simulink model "momentumBasedFlightSim"  (R2022a)
settings: Solver=FixedStepDiscrete  StartTime=0.0  StopTime=Config.simulationTime  FixedStep=Config.tStep  RelTol=1e-3
InitFcn:
  | cd(fileparts(which(bdroot)));
  | initMomentumBasedFlight;
StopFcn:
  | cd(fileparts(which(bdroot)));
  | stopMomentumBasedFlight;
undefined symbols (not defined in the file or in its folder): Config, DiscIntNeverNeededParam
libraries: WBToolboxLibrary x31, cstblocks x3, momentum_flight_control_sublib x2, thrust_estimation_sublib x1, jets_control x1
(part 2 of 2)

== system momentumBasedFlightSim/FLIGHT CONTROLLER (CORE) V6.0/FLIGHT CONTROL/Momentum-based Flight Control QP/Filtering and Saturations/Filters on jointVel ==
  jointVel_star_QP : Inport
  Compare_filtered_jointVel : Scope  NumInputPorts=2
  Constant : Constant  Value=ones(4,1)*11
  Constant1 : Constant  Value=Config.BALANCING_NO_JETS
  Constant2 : Constant  Value=Config.filter.cutOffFrequency
  Constant3 : Constant  Value=Config.FILTER_SDOT_AFTER_QP
  Dead Zone1 : DeadZone  LowerValue=-Config.deadzone.jointVel_deadzone  UpperValue=Config.deadzone.jointVel_deadzone
  Discrete Varying Lowpass1 : cstblocks/Linear Parameter Varying/Discrete Varying Lowpass  N=2  w0=0  Ts=Config.tStep
      settings: SourceProductBaseCode=CT
  Saturation1 : Saturate  UpperLimit=Config.saturation.maxJointVelDes  LowerLimit=-Config.saturation.maxJointVelDes
  Switch : Switch  Criteria=u2 > Threshold  SaturateOnIntegerOverflow=off  InputSameDT=off
  Switch1 : Switch  Criteria=u2 > Threshold  SaturateOnIntegerOverflow=off  InputSameDT=off
  joint_vel_saturation : MATLAB Function  TreatAsAtomicUnit=on
  jointVel_star_filt : Outport  VectorParamsAs1DForOutWhenUnconnected=off
  tag scope: JointVelocityDesired=global
  wires:
  Constant3/1 -> Switch1/2
  Switch1/1 -> jointVel_star_filt/1
  joint_vel_saturation/1(jointVel) -> Switch1/1, Compare_filtered_jointVel/1
  Constant2/1 -> Discrete Varying Lowpass1/2
  Saturation1/1 -> joint_vel_saturation/2(jointVel_des)
  Discrete Varying Lowpass1/1 -> Dead Zone1/1
  Dead Zone1/1 -> Saturation1/1
  jointVel_star_QP/1 -> Discrete Varying Lowpass1/1, Switch1/3, Compare_filtered_jointVel/2, [JointVelocityDesired]
  Switch/1 -> joint_vel_saturation/3(JetState)
  Constant1/1 -> Switch/2
  [JetLog] -> Switch/3
  Constant/1 -> Switch/1
  [jointPos_meas] -> joint_vel_saturation/1(jointPos)

== system momentumBasedFlightSim/FLIGHT CONTROLLER (CORE) V6.0/FLIGHT CONTROL/Flight 0 Reference Generator/Compute Gains And References/Online Planner/Smooth CoM References ==
  posCoM_des : Inport
  accCoM_gravity_ref : Inport  Port=2
  Combine CoM References : MATLAB Function  TreatAsAtomicUnit=on
  MatchSignalSizes{,1..3} (4 alike) : WBToolboxLibrary/Utilities/MatchSignalSizes
      settings: SourceProductName=WholeBodyToolbox
  MinimumJerkTrajectoryGenerator : WBToolboxLibrary/Utilities/MinimumJerkTrajectoryGenerator  externalSettlingTime=off  settlingTime=Config.planner.timeToReachHovering  sampleTime=Config.tStep  resetOnSettlingTime=off  firstDerivatives=off  secondDerivatives=off  explicitInitialValue=off
      settings: SourceProductName=WholeBodyToolbox
  MinimumJerkTrajectoryGenerator1 : WBToolboxLibrary/Utilities/MinimumJerkTrajectoryGenerator  externalSettlingTime=off  settlingTime=Config.planner.smoothingTimeCoMRef  sampleTime=Config.tStep  resetOnSettlingTime=off  firstDerivatives=on  secondDerivatives=on  explicitInitialValue=off
      settings: SourceProductName=WholeBodyToolbox
  pos_vel_acc_jerk_CoM_des : Outport  VectorParamsAs1DForOutWhenUnconnected=off
  wires:
  MinimumJerkTrajectoryGenerator/1 -> MatchSignalSizes3/2
  MinimumJerkTrajectoryGenerator1/3 -> MatchSignalSizes2/2
  MinimumJerkTrajectoryGenerator1/2 -> MatchSignalSizes1/2
  posCoM_des/1 -> MinimumJerkTrajectoryGenerator1/1, MatchSignalSizes1/1, MatchSignalSizes2/1, MatchSignalSizes3/1, MatchSignalSizes/1
  MatchSignalSizes1/1 -> Combine CoM References/2(CoM_vel)
  MatchSignalSizes2/1 -> Combine CoM References/3(CoM_acc)
  MatchSignalSizes3/1 -> Combine CoM References/4(CoM_acc_gravity)
  MatchSignalSizes/1 -> Combine CoM References/1(CoM_pos)
  MinimumJerkTrajectoryGenerator1/1 -> MatchSignalSizes/2
  accCoM_gravity_ref/1 -> MinimumJerkTrajectoryGenerator/1
  Combine CoM References/1(pos_vel_acc_jerk_CoM_des) -> pos_vel_acc_jerk_CoM_des/1

== system momentumBasedFlightSim/FLIGHT CONTROLLER (CORE) V6.0/FLIGHT CONTROL/Momentum-based Flight Control QP/Compute QP Quantities/Integrate CoM Velocity/Get CoM Position Error from Integral ==
  kinematics : Inport
  systemState : Inport  Port=2
  gainsAndReferences : Inport  Port=3
  Bus Selector : BusSelector  OutputSignals=stateVel
  Bus Selector1 : BusSelector  OutputSignals=pos_vel_acc_jerk_CoM_des
  Bus Selector2 : BusSelector  OutputSignals=J_CoM
  Constant : Constant  Value=zeros(3,1)
  Dead Zone : DeadZone  LowerValue=-Config.deadzone.velCoM_deadzone  UpperValue=Config.deadzone.velCoM_deadzone
  Integrate velCoM_error : DiscreteIntegrator  InitialConditionSource=external  SampleTime=Config.tStep  ICPrevOutput=DiscIntNeverNeededParam  ICPrevScaledInput=DiscIntNeverNeededParam
  MatrixMultiply : Product  Multiplication=Matrix(*)
  Selector1 : Selector  NumberOfDimensions=2  InputPortWidth=3  IndexOptions=Index vector (dialog),Index vector (dialog)  Indices=[1 2 3],2  OutputSizes=1,1
  Sum1 : Sum  Inputs=|+-
  posCoM_error_fromIntegral : Outport
  wires:
  Bus Selector2/1 -> MatrixMultiply/1  "<J_CoM>"
  Selector1/1 -> Sum1/2  "velCoM_des"
  MatrixMultiply/1 -> Sum1/1  "velCoM"
  Integrate velCoM_error/1 -> posCoM_error_fromIntegral/1
  Bus Selector1/1 -> Selector1/1  "<pos_vel_acc_jerk_CoM_des>"
  gainsAndReferences/1 -> Bus Selector1/1
  systemState/1 -> Bus Selector/1
  Sum1/1 -> Dead Zone/1
  kinematics/1 -> Bus Selector2/1
  Bus Selector/1 -> MatrixMultiply/2  "<stateVel>"
  Constant/1 -> Integrate velCoM_error/2
  Dead Zone/1 -> Integrate velCoM_error/1

== system momentumBasedFlightSim/FLIGHT CONTROLLER (CORE) V6.0/FLIGHT CONTROL/Momentum-based Flight Control QP/Compute QP Quantities/Integrate CoM Velocity/Get CoM Position Error from Integral but Only in Hovering ==
  feetContactIsActive : Inport
  kinematics : Inport  Port=2
  systemState : Inport  Port=3
  gainsAndReferences : Inport  Port=4
  Bus Selector : BusSelector  OutputSignals=stateVel
  Bus Selector1 : BusSelector  OutputSignals=pos_vel_acc_jerk_CoM_des
  Bus Selector2 : BusSelector  OutputSignals=posCoM,J_CoM
  Dead Zone : DeadZone  LowerValue=-Config.deadzone.velCoM_deadzone  UpperValue=Config.deadzone.velCoM_deadzone
  Get CoM initial condition : MATLAB Function  TreatAsAtomicUnit=on
  Integrate velCoM_error : DiscreteIntegrator  ExternalReset=either  InitialConditionSource=external  SampleTime=Config.tStep  ICPrevOutput=DiscIntNeverNeededParam  ICPrevScaledInput=DiscIntNeverNeededParam
  MatrixMultiply : Product  Multiplication=Matrix(*)
  Selector1 : Selector  NumberOfDimensions=2  InputPortWidth=3  IndexOptions=Index vector (dialog),Index vector (dialog)  Indices=[1 2 3],2  OutputSizes=1,1
  Selector2 : Selector  NumberOfDimensions=2  InputPortWidth=3  IndexOptions=Index vector (dialog),Index vector (dialog)  Indices=[1 2 3],1  OutputSizes=1,1
  Sum1 : Sum  Inputs=|+-
  Sum2 : Sum  Inputs=|+-
  Switch : Switch  Criteria=u2 > Threshold  SaturateOnIntegerOverflow=off  InputSameDT=off
  posCoM_error_fromInt_HoveringOnly : Outport
  wires:
  Get CoM initial condition/1(error_posCoM_0) -> Integrate velCoM_error/3
  Bus Selector2/2 -> MatrixMultiply/1  "<J_CoM>"
  Selector1/1 -> Sum1/2  "velCoM_des"
  MatrixMultiply/1 -> Sum1/1  "velCoM"
  Bus Selector1/1 -> Selector2/1, Selector1/1  "<pos_vel_acc_jerk_CoM_des>"
  gainsAndReferences/1 -> Bus Selector1/1
  systemState/1 -> Bus Selector/1
  Sum1/1 -> Dead Zone/1
  kinematics/1 -> Bus Selector2/1
  Bus Selector/1 -> MatrixMultiply/2  "<stateVel>"
  Sum2/1 -> Get CoM initial condition/2(error_posCoM), Switch/1
  Switch/1 -> posCoM_error_fromInt_HoveringOnly/1
  Bus Selector2/1 -> Sum2/1  "<posCoM>"
  Selector2/1 -> Sum2/2  "posCoM_des"
  Integrate velCoM_error/1 -> Switch/3
  feetContactIsActive/1 -> Switch/2, Integrate velCoM_error/2, Get CoM initial condition/1(feetContactIsActive)
  Dead Zone/1 -> Integrate velCoM_error/1

== system momentumBasedFlightSim/FLIGHT CONTROLLER (CORE) V6.0/FLIGHT CONTROL/Momentum-based Flight Control QP/Compute QP Quantities/Integrate CoM Velocity/Get CoM Position Error from Kinematics ==
  kinematics : Inport
  gainsAndReferences : Inport  Port=2
  Bus Selector1 : BusSelector  OutputSignals=pos_vel_acc_jerk_CoM_des
  Bus Selector2 : BusSelector  OutputSignals=posCoM
  Selector1 : Selector  NumberOfDimensions=2  InputPortWidth=3  IndexOptions=Index vector (dialog),Index vector (dialog)  Indices=[1 2 3],1  OutputSizes=1,1
  Sum1 : Sum  Inputs=|+-
  posCoM_error_fromKinematics : Outport
  wires:
  Bus Selector2/1 -> Sum1/1  "<posCoM>"
  Selector1/1 -> Sum1/2  "posCoM_des"
  Sum1/1 -> posCoM_error_fromKinematics/1
  Bus Selector1/1 -> Selector1/1  "<pos_vel_acc_jerk_CoM_des>"
  gainsAndReferences/1 -> Bus Selector1/1
  kinematics/1 -> Bus Selector2/1

== system momentumBasedFlightSim/FLIGHT CONTROLLER (CORE) V6.0/FLIGHT CONTROL/Momentum-based Flight Control QP/Compute QP Quantities/Integrate CoM Velocity/Select CoM Pos Error ==
  feetContactIsActive : Inport
  posCoM_error_fromInt_HoveringOnly : Inport  Port=2
  posCoM_error_fromIntegral : Inport  Port=3
  posCoM_error_fromKinematics : Inport  Port=4
  CoM Pos Errors : Scope  NumInputPorts=4
  Select CoM Pos Error : MATLAB Function  TreatAsAtomicUnit=on
  posCoM_error : Outport
  wires:
  posCoM_error_fromKinematics/1 -> CoM Pos Errors/3, Select CoM Pos Error/3(posCoM_error_fromKinematics)  "posCoM_error_fromKinematics"
  posCoM_error_fromIntegral/1 -> Select CoM Pos Error/2(posCoM_error_fromIntegral), CoM Pos Errors/2  "posCoM_error_fromIntegral"
  posCoM_error_fromInt_HoveringOnly/1 -> CoM Pos Errors/1, Select CoM Pos Error/1(posCoM_error_fromInt_HoveringOnly)  "posCoM_error_fromInt_HoveringOnly"
  Select CoM Pos Error/1(posCoM_error) -> posCoM_error/1
  feetContactIsActive/1 -> CoM Pos Errors/4  "robotIsBalancing"

== system momentumBasedFlightSim/FLIGHT CONTROLLER (CORE) V6.0/FLIGHT CONTROL/Momentum-based Flight Control QP/Compute QP Quantities/Visualize QP Quantities/Cost Function ==
  uStar : Inport
  Hessian : Inport  Port=2
  gradient : Inport  Port=3
  costVectorQP : Inport  Port=4
  Add1 : Sum
  Demux : Demux  Outputs=8
  Full Cost Check : Scope
  Gain : Gain  Gain=0.5
  Matrix Multiply : Product  Multiplication=Matrix(*)
  Matrix Multiply1 : Product  Multiplication=Matrix(*)
  Matrix Multiply2 : Product  Multiplication=Matrix(*)
  Transpose : Math  Operator=transpose
  costs in QP function : Scope  NumInputPorts=8
  wires:
  Demux/1 -> costs in QP function/1  "linMom_xy"
  Gain/1 -> Add1/2  "(uT * H * u) / 2"
  Add1/1 -> Full Cost Check/1  "(uT * H * u)/2 + uT * g"
  gradient/1 -> Matrix Multiply2/2
  Matrix Multiply2/1 -> Add1/1  "uT * g"
  Matrix Multiply1/1 -> Gain/1
  Matrix Multiply/1 -> Matrix Multiply1/1
  Hessian/1 -> Matrix Multiply/2
  Transpose/1 -> Matrix Multiply/1, Matrix Multiply2/1
  uStar/1 -> Transpose/1, Matrix Multiply1/2
  Demux/7 -> costs in QP function/7  "TDotPost"
  Demux/6 -> costs in QP function/6  "legsPost"
  Demux/5 -> costs in QP function/5  "armsPost"
  Demux/2 -> costs in QP function/2  "linMom_z"
  Demux/8 -> costs in QP function/8  "symmTDot"
  Demux/3 -> costs in QP function/3  "angMom"
  Demux/4 -> costs in QP function/4  "torsoPost"
  costVectorQP/1 -> Demux/1

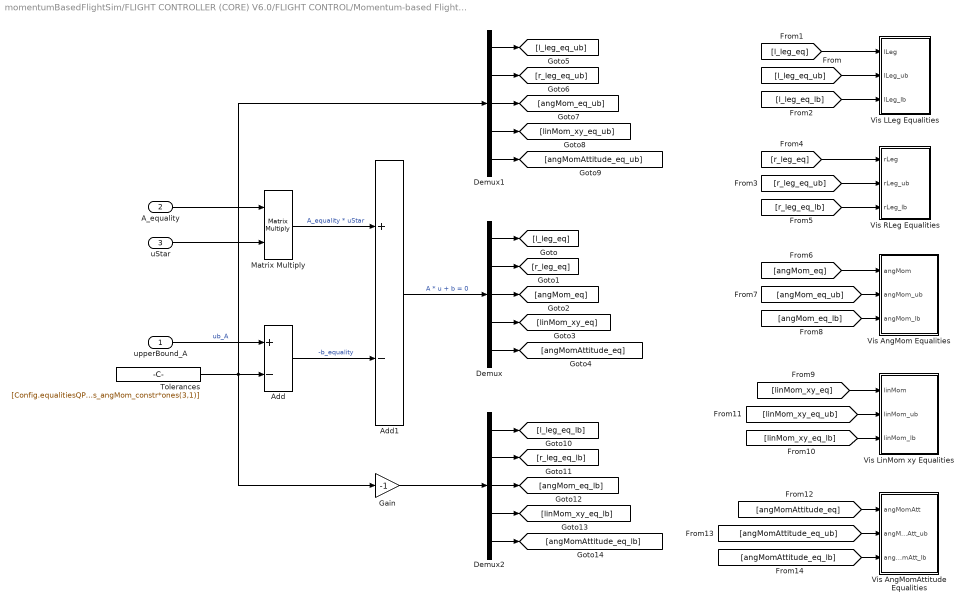
== system momentumBasedFlightSim/FLIGHT CONTROLLER (CORE) V6.0/FLIGHT CONTROL/Momentum-based Flight Control QP/Compute QP Quantities/Visualize QP Quantities/Equality Constraints ==
  upperBound_A : Inport
  A_equality : Inport  Port=2
  uStar : Inport  Port=3
  Add : Sum  Inputs=+-
  Add1 : Sum  Inputs=+-
  Demux : Demux  Outputs=[Config.N_LEGS/2; Config.N_LEGS/2; 3; 2; 3]
  Demux1 : Demux  Outputs=[Config.N_LEGS/2; Config.N_LEGS/2; 3; 2; 3]
  Demux2 : Demux  Outputs=[Config.N_LEGS/2; Config.N_LEGS/2; 3; 2; 3]
  Gain : Gain  Gain=-1
  Matrix Multiply : Product  Multiplication=Matrix(*)
  Tolerances : Constant  Value=[Config.equalitiesQP.eps_legs*ones(Config.N_LEGS,1); Config.equalitiesQP.eps_angMom*ones(3,1); Config.equalitiesQP.eps_linMom_xy*ones(2,1); Config.equalitiesQP.eps_angMom_constr*ones(3,1)]
  Vis AngMom Equalities : Subsystem
  Vis AngMomAttitude Equalities : Subsystem
  Vis LLeg Equalities : Subsystem
  Vis LinMom xy Equalities : Subsystem
  Vis RLeg Equalities : Subsystem
  wires:
  [angMomAttitude_eq_lb] -> Vis AngMomAttitude Equalities/3(angMomAtt_lb)
  [angMomAttitude_eq_ub] -> Vis AngMomAttitude Equalities/2(angMomAtt_ub)
  [angMomAttitude_eq] -> Vis AngMomAttitude Equalities/1(angMomAtt)
  [linMom_xy_eq] -> Vis LinMom xy Equalities/1(linMom)
  [linMom_xy_eq_ub] -> Vis LinMom xy Equalities/2(linMom_ub)
  [linMom_xy_eq_lb] -> Vis LinMom xy Equalities/3(linMom_lb)
  [angMom_eq_lb] -> Vis AngMom Equalities/3(angMom_lb)
  [angMom_eq_ub] -> Vis AngMom Equalities/2(angMom_ub)
  [angMom_eq] -> Vis AngMom Equalities/1(angMom)
  [r_leg_eq_lb] -> Vis RLeg Equalities/3(rLeg_lb)
  [r_leg_eq] -> Vis RLeg Equalities/1(rLeg)
  [r_leg_eq_ub] -> Vis RLeg Equalities/2(rLeg_ub)
  [l_leg_eq_lb] -> Vis LLeg Equalities/3(lLeg_lb)
  [l_leg_eq_ub] -> Vis LLeg Equalities/2(lLeg_ub)
  [l_leg_eq] -> Vis LLeg Equalities/1(lLeg)
  Demux2/1 -> [l_leg_eq_lb]
  Demux2/2 -> [r_leg_eq_lb]
  Demux2/5 -> [angMomAttitude_eq_lb]
  Demux2/4 -> [linMom_xy_eq_lb]
  Demux2/3 -> [angMom_eq_lb]
  Demux1/4 -> [linMom_xy_eq_ub]
  Demux1/2 -> [r_leg_eq_ub]
  Demux1/1 -> [l_leg_eq_ub]
  Demux1/3 -> [angMom_eq_ub]
  Demux1/5 -> [angMomAttitude_eq_ub]
  Demux/5 -> [angMomAttitude_eq]
  Demux/4 -> [linMom_xy_eq]
  Demux/3 -> [angMom_eq]
  Demux/2 -> [r_leg_eq]
  Demux/1 -> [l_leg_eq]
  Tolerances/1 -> Demux1/1, Gain/1, Add/2
  Add1/1 -> Demux/1  "A * u + b = 0"
  Matrix Multiply/1 -> Add1/1  "A_equality * uStar"
  uStar/1 -> Matrix Multiply/2
  A_equality/1 -> Matrix Multiply/1
  Add/1 -> Add1/2  "-b_equality"
  upperBound_A/1 -> Add/1  "ub_A"
  Gain/1 -> Demux2/1

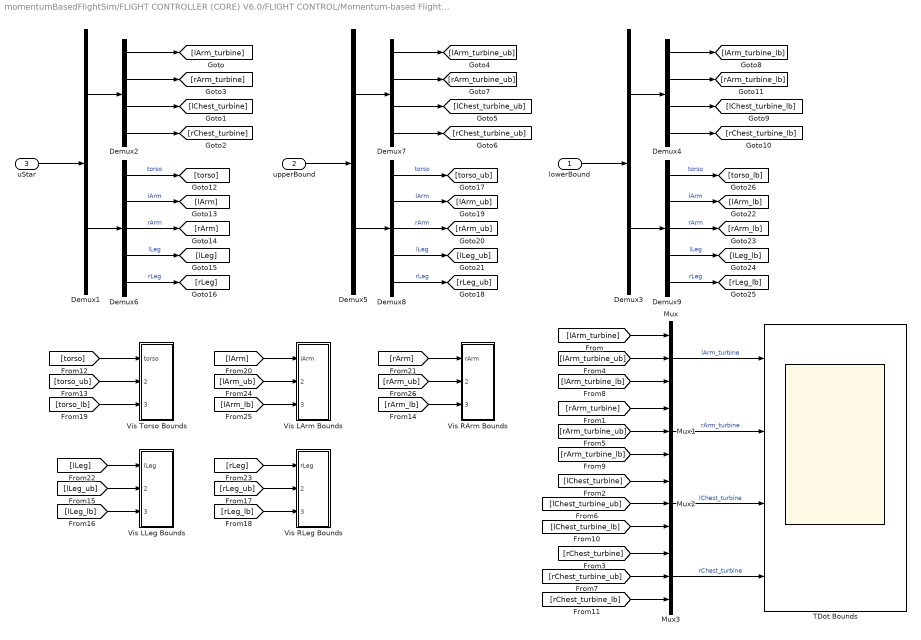
== system momentumBasedFlightSim/FLIGHT CONTROLLER (CORE) V6.0/FLIGHT CONTROL/Momentum-based Flight Control QP/Compute QP Quantities/Visualize QP Quantities/Input Boundaries ==
  lowerBound : Inport
  upperBound : Inport  Port=2
  uStar : Inport  Port=3
  Demux1 : Demux  Outputs=[Config.N_JETS; Config.N_DOF]
  Demux2 : Demux  Outputs=Config.N_JETS
  Demux3 : Demux  Outputs=[Config.N_JETS; Config.N_DOF]
  Demux4 : Demux  Outputs=Config.N_JETS
  Demux5 : Demux  Outputs=[Config.N_JETS; Config.N_DOF]
  Demux6 : Demux  Outputs=Config.numOfJointsForEachControlboard
  Demux7 : Demux  Outputs=Config.N_JETS
  Demux8 : Demux  Outputs=Config.numOfJointsForEachControlboard
  Demux9 : Demux  Outputs=Config.numOfJointsForEachControlboard
  Mux{,1..3} (4 alike) : Mux  Inputs=3
  TDot Bounds : Scope  NumInputPorts=4
  Vis LArm Bounds : Subsystem
  Vis LLeg Bounds : Subsystem
  Vis RArm Bounds : Subsystem
  Vis RLeg Bounds : Subsystem
  Vis Torso Bounds : Subsystem
  wires:
  Mux3/1 -> TDot Bounds/4  "rChest_turbine"
  Mux2/1 -> TDot Bounds/3  "lChest_turbine"
  Mux1/1 -> TDot Bounds/2  "rArm_turbine"
  Mux/1 -> TDot Bounds/1  "lArm_turbine"
  [torso_lb] -> Vis Torso Bounds/3(torso_lb)
  [torso_ub] -> Vis Torso Bounds/2(torso_ub)
  [torso] -> Vis Torso Bounds/1(torso)
  [lLeg] -> Vis LLeg Bounds/1(lLeg)
  [lArm_ub] -> Vis LArm Bounds/2(lArm_ub)
  [lLeg_lb] -> Vis LLeg Bounds/3(lLeg_lb)
  [lArm_lb] -> Vis LArm Bounds/3(lArm_lb)
  [rArm_lb] -> Vis RArm Bounds/3(rArm_lb)
  [rLeg_ub] -> Vis RLeg Bounds/2(rLeg_ub)
  [rArm] -> Vis RArm Bounds/1(rArm)
  [lArm] -> Vis LArm Bounds/1(lArm)
  [rArm_ub] -> Vis RArm Bounds/2(rArm_ub)
  [lLeg_ub] -> Vis LLeg Bounds/2(lLeg_ub)
  [rLeg_lb] -> Vis RLeg Bounds/3(rLeg_lb)
  [rLeg] -> Vis RLeg Bounds/1(rLeg)
  Demux9/5 -> [rLeg_lb]  "rLeg"
  Demux3/1 -> Demux4/1
  lowerBound/1 -> Demux3/1
  Demux4/3 -> [lChest_turbine_lb]
  Demux9/1 -> [torso_lb]  "torso"
  Demux9/2 -> [lArm_lb]  "lArm"
  Demux9/4 -> [lLeg_lb]  "lLeg"
  Demux4/2 -> [rArm_turbine_lb]
  Demux4/1 -> [lArm_turbine_lb]
  Demux3/2 -> Demux9/1
  Demux9/3 -> [rArm_lb]  "rArm"
  Demux4/4 -> [rChest_turbine_lb]
  upperBound/1 -> Demux5/1
  Demux7/1 -> [lArm_turbine_ub]
  Demux7/4 -> [rChest_turbine_ub]
  Demux8/4 -> [lLeg_ub]  "lLeg"
  Demux7/2 -> [rArm_turbine_ub]
  Demux5/2 -> Demux8/1
  Demux8/5 -> [rLeg_ub]  "rLeg"
  Demux8/3 -> [rArm_ub]  "rArm"
  Demux8/2 -> [lArm_ub]  "lArm"
  Demux5/1 -> Demux7/1
  Demux8/1 -> [torso_ub]  "torso"
  Demux7/3 -> [lChest_turbine_ub]
  Demux6/4 -> [lLeg]  "lLeg"
  Demux6/1 -> [torso]  "torso"
  Demux1/2 -> Demux6/1
  Demux6/5 -> [rLeg]  "rLeg"
  Demux6/2 -> [lArm]  "lArm"
  Demux6/3 -> [rArm]  "rArm"
  Demux2/4 -> [rChest_turbine]
  [rChest_turbine_ub] -> Mux3/2
  [lChest_turbine_lb] -> Mux2/3
  [lChest_turbine] -> Mux2/1
  Demux1/1 -> Demux2/1
  [rArm_turbine_lb] -> Mux1/3
  Demux2/3 -> [lChest_turbine]
  [lArm_turbine] -> Mux/1
  Demux2/2 -> [rArm_turbine]
  [rArm_turbine] -> Mux1/1
  [lChest_turbine_ub] -> Mux2/2
  [rChest_turbine_lb] -> Mux3/3
  [rArm_turbine_ub] -> Mux1/2
  [lArm_turbine_lb] -> Mux/3
  [lArm_turbine_ub] -> Mux/2
  Demux2/1 -> [lArm_turbine]
  [rChest_turbine] -> Mux3/1
  uStar/1 -> Demux1/1

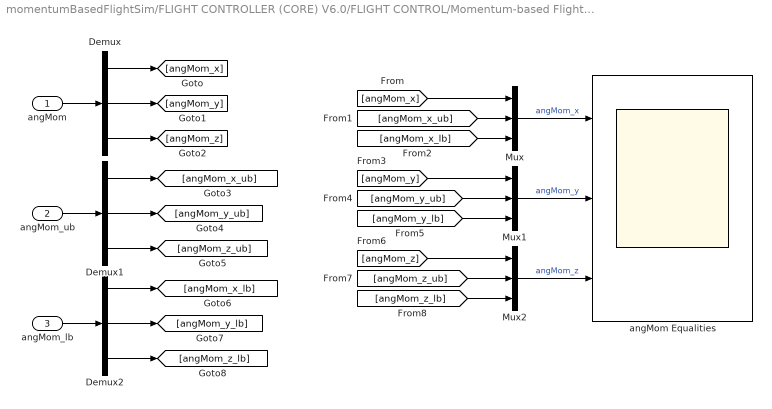
== system momentumBasedFlightSim/FLIGHT CONTROLLER (CORE) V6.0/FLIGHT CONTROL/Momentum-based Flight Control QP/Compute QP Quantities/Visualize QP Quantities/Equality Constraints/Vis AngMom Equalities ==
  angMom : Inport
  angMom_ub : Inport  Port=2
  angMom_lb : Inport  Port=3
  Demux : Demux  Outputs=3
  Demux1 : Demux  Outputs=3
  Demux2 : Demux  Outputs=3
  Mux : Mux  Inputs=3
  Mux1 : Mux  Inputs=3
  Mux2 : Mux  Inputs=3
  angMom Equalities : Scope  NumInputPorts=3
  wires:
  [angMom_z] -> Mux2/1
  [angMom_y] -> Mux1/1
  [angMom_x] -> Mux/1
  Mux1/1 -> angMom Equalities/2  "angMom_y"
  Mux2/1 -> angMom Equalities/3  "angMom_z"
  Mux/1 -> angMom Equalities/1  "angMom_x"
  [angMom_z_lb] -> Mux2/3
  [angMom_z_ub] -> Mux2/2
  [angMom_y_ub] -> Mux1/2
  [angMom_y_lb] -> Mux1/3
  [angMom_x_lb] -> Mux/3
  [angMom_x_ub] -> Mux/2
  Demux2/3 -> [angMom_z_lb]
  Demux2/2 -> [angMom_y_lb]
  Demux2/1 -> [angMom_x_lb]
  Demux1/3 -> [angMom_z_ub]
  Demux1/1 -> [angMom_x_ub]
  Demux1/2 -> [angMom_y_ub]
  Demux/3 -> [angMom_z]
  Demux/2 -> [angMom_y]
  Demux/1 -> [angMom_x]
  angMom_lb/1 -> Demux2/1
  angMom_ub/1 -> Demux1/1
  angMom/1 -> Demux/1

== system momentumBasedFlightSim/FLIGHT CONTROLLER (CORE) V6.0/FLIGHT CONTROL/Momentum-based Flight Control QP/Compute QP Quantities/Visualize QP Quantities/Equality Constraints/Vis AngMomAttitude Equalities ==
  angMomAtt : Inport
  angMomAtt_ub : Inport  Port=2
  angMomAtt_lb : Inport  Port=3
  Demux : Demux  Outputs=3
  Demux1 : Demux  Outputs=3
  Demux2 : Demux  Outputs=3
  Mux : Mux  Inputs=3
  Mux1 : Mux  Inputs=3
  Mux2 : Mux  Inputs=3
  angMomAtt Equalities : Scope  NumInputPorts=3
  wires:
  [angMom_z] -> Mux2/1
  [angMom_y] -> Mux1/1
  [angMom_x] -> Mux/1
  Mux1/1 -> angMomAtt Equalities/2  "angMomAtt_y"
  Mux2/1 -> angMomAtt Equalities/3  "angMomAtt_z"
  Mux/1 -> angMomAtt Equalities/1  "angMomAtt_x"
  [angMom_z_lb] -> Mux2/3
  [angMom_z_ub] -> Mux2/2
  [angMom_y_ub] -> Mux1/2
  [angMom_y_lb] -> Mux1/3
  [angMom_x_lb] -> Mux/3
  [angMom_x_ub] -> Mux/2
  Demux2/3 -> [angMom_z_lb]
  Demux2/2 -> [angMom_y_lb]
  Demux2/1 -> [angMom_x_lb]
  Demux1/3 -> [angMom_z_ub]
  Demux1/1 -> [angMom_x_ub]
  Demux1/2 -> [angMom_y_ub]
  Demux/3 -> [angMom_z]
  Demux/2 -> [angMom_y]
  Demux/1 -> [angMom_x]
  angMomAtt_lb/1 -> Demux2/1
  angMomAtt_ub/1 -> Demux1/1
  angMomAtt/1 -> Demux/1

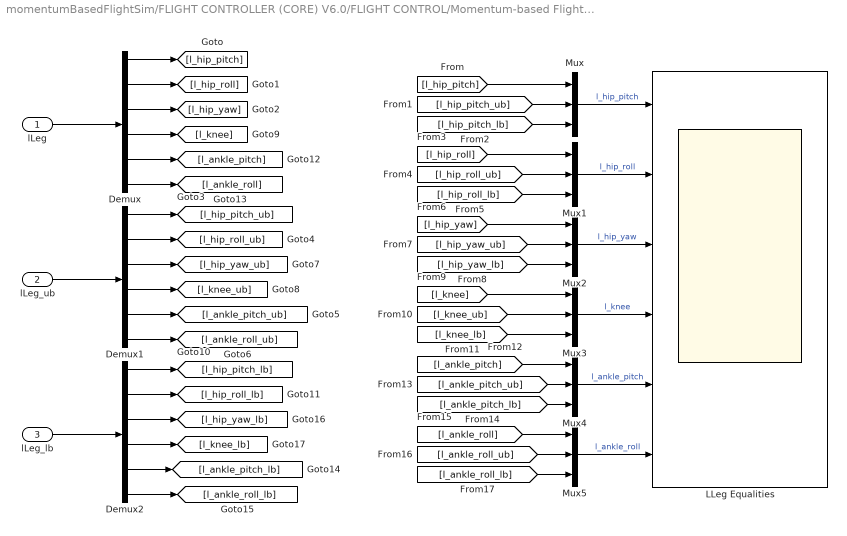
== system momentumBasedFlightSim/FLIGHT CONTROLLER (CORE) V6.0/FLIGHT CONTROL/Momentum-based Flight Control QP/Compute QP Quantities/Visualize QP Quantities/Equality Constraints/Vis LLeg Equalities ==
  lLeg : Inport
  lLeg_ub : Inport  Port=2
  lLeg_lb : Inport  Port=3
  Demux : Demux  Outputs=Config.N_LEGS/2
  Demux1 : Demux  Outputs=Config.N_LEGS/2
  Demux2 : Demux  Outputs=Config.N_LEGS/2
  LLeg Equalities : Scope  NumInputPorts=6
  Mux{,1..5} (6 alike) : Mux  Inputs=3
  wires:
  [l_ankle_roll_lb] -> Mux5/3
  [l_ankle_roll_ub] -> Mux5/2
  [l_ankle_roll] -> Mux5/1
  [l_ankle_pitch_lb] -> Mux4/3
  [l_ankle_pitch_ub] -> Mux4/2
  [l_ankle_pitch] -> Mux4/1
  [l_knee_lb] -> Mux3/3
  [l_knee_ub] -> Mux3/2
  [l_knee] -> Mux3/1
  [l_hip_yaw_lb] -> Mux2/3
  [l_hip_yaw_ub] -> Mux2/2
  [l_hip_yaw] -> Mux2/1
  [l_hip_roll_lb] -> Mux1/3
  [l_hip_roll_ub] -> Mux1/2
  [l_hip_roll] -> Mux1/1
  [l_hip_pitch_lb] -> Mux/3
  [l_hip_pitch_ub] -> Mux/2
  [l_hip_pitch] -> Mux/1
  Mux5/1 -> LLeg Equalities/6  "l_ankle_roll"
  Mux4/1 -> LLeg Equalities/5  "l_ankle_pitch"
  Demux2/4 -> [l_knee_lb]
  Demux2/3 -> [l_hip_yaw_lb]
  Demux2/1 -> [l_hip_pitch_lb]
  Demux2/2 -> [l_hip_roll_lb]
  Demux2/5 -> [l_ankle_pitch_lb]
  Demux2/6 -> [l_ankle_roll_lb]
  lLeg_lb/1 -> Demux2/1
  Demux1/1 -> [l_hip_pitch_ub]
  Demux1/2 -> [l_hip_roll_ub]
  Demux1/5 -> [l_ankle_pitch_ub]
  lLeg_ub/1 -> Demux1/1
  Demux1/6 -> [l_ankle_roll_ub]
  Demux1/4 -> [l_knee_ub]
  Demux1/3 -> [l_hip_yaw_ub]
  Demux/6 -> [l_ankle_roll]
  Demux/5 -> [l_ankle_pitch]
  Mux1/1 -> LLeg Equalities/2  "l_hip_roll"
  Mux2/1 -> LLeg Equalities/3  "l_hip_yaw"
  Demux/1 -> [l_hip_pitch]
  Demux/3 -> [l_hip_yaw]
  Mux3/1 -> LLeg Equalities/4  "l_knee"
  Demux/2 -> [l_hip_roll]
  Demux/4 -> [l_knee]
  lLeg/1 -> Demux/1
  Mux/1 -> LLeg Equalities/1  "l_hip_pitch"

== system momentumBasedFlightSim/FLIGHT CONTROLLER (CORE) V6.0/FLIGHT CONTROL/Momentum-based Flight Control QP/Compute QP Quantities/Visualize QP Quantities/Equality Constraints/Vis LinMom xy Equalities ==
  linMom : Inport
  linMom_ub : Inport  Port=2
  linMom_lb : Inport  Port=3
  Demux : Demux  Outputs=2
  Demux1 : Demux  Outputs=2
  Demux2 : Demux  Outputs=2
  Mux : Mux  Inputs=3
  Mux1 : Mux  Inputs=3
  linMom_xy Equalities : Scope  NumInputPorts=2
  wires:
  [linMom_y] -> Mux1/1
  [linMom_x] -> Mux/1
  Mux1/1 -> linMom_xy Equalities/2  "linMom_y"
  Mux/1 -> linMom_xy Equalities/1  "linMom_x"
  [linMom_y_ub] -> Mux1/2
  [linMom_y_lb] -> Mux1/3
  [linMom_x_lb] -> Mux/3
  [linMom_x_ub] -> Mux/2
  Demux2/2 -> [linMom_y_lb]
  Demux2/1 -> [linMom_x_lb]
  Demux1/1 -> [linMom_x_ub]
  Demux1/2 -> [linMom_y_ub]
  Demux/2 -> [linMom_y]
  Demux/1 -> [linMom_x]
  linMom_lb/1 -> Demux2/1
  linMom_ub/1 -> Demux1/1
  linMom/1 -> Demux/1

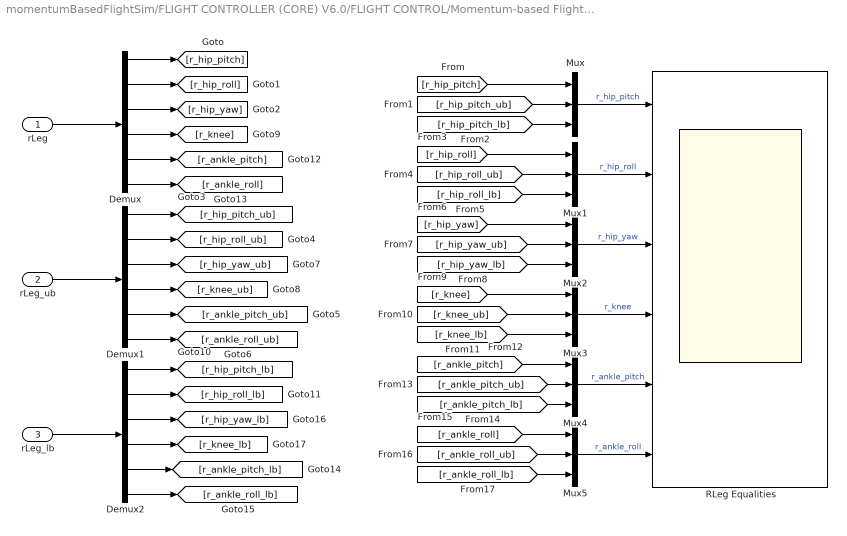
== system momentumBasedFlightSim/FLIGHT CONTROLLER (CORE) V6.0/FLIGHT CONTROL/Momentum-based Flight Control QP/Compute QP Quantities/Visualize QP Quantities/Equality Constraints/Vis RLeg Equalities ==
  rLeg : Inport
  rLeg_ub : Inport  Port=2
  rLeg_lb : Inport  Port=3
  Demux : Demux  Outputs=Config.N_LEGS/2
  Demux1 : Demux  Outputs=Config.N_LEGS/2
  Demux2 : Demux  Outputs=Config.N_LEGS/2
  Mux{,1..5} (6 alike) : Mux  Inputs=3
  RLeg Equalities : Scope  NumInputPorts=6
  wires:
  Demux/2 -> [r_hip_roll]
  Demux1/4 -> [r_knee_ub]
  Mux2/1 -> RLeg Equalities/3  "r_hip_yaw"
  Demux1/2 -> [r_hip_roll_ub]
  Demux1/5 -> [r_ankle_pitch_ub]
  [r_ankle_pitch_lb] -> Mux4/3
  [r_hip_yaw_lb] -> Mux2/3
  Demux1/6 -> [r_ankle_roll_ub]
  [r_hip_roll] -> Mux1/1
  Demux1/3 -> [r_hip_yaw_ub]
  Demux1/1 -> [r_hip_pitch_ub]
  [r_ankle_pitch] -> Mux4/1
  Demux/1 -> [r_hip_pitch]
  [r_knee] -> Mux3/1
  Demux/4 -> [r_knee]
  Mux4/1 -> RLeg Equalities/5  "r_ankle_pitch"
  [r_hip_pitch] -> Mux/1
  Demux2/5 -> [r_ankle_pitch_lb]
  Demux2/3 -> [r_hip_yaw_lb]
  Demux2/2 -> [r_hip_roll_lb]
  [r_ankle_roll_lb] -> Mux5/3
  [r_hip_yaw_ub] -> Mux2/2
  [r_hip_yaw] -> Mux2/1
  [r_hip_pitch_lb] -> Mux/3
  Demux/6 -> [r_ankle_roll]
  rLeg/1 -> Demux/1
  Demux2/1 -> [r_hip_pitch_lb]
  [r_knee_lb] -> Mux3/3
  Mux3/1 -> RLeg Equalities/4  "r_knee"
  Mux1/1 -> RLeg Equalities/2  "r_hip_roll"
  Demux2/4 -> [r_knee_lb]
  [r_knee_ub] -> Mux3/2
  [r_ankle_roll] -> Mux5/1
  [r_hip_roll_lb] -> Mux1/3
  [r_hip_roll_ub] -> Mux1/2
  [r_ankle_roll_ub] -> Mux5/2
  rLeg_ub/1 -> Demux1/1
  [r_hip_pitch_ub] -> Mux/2
  Mux5/1 -> RLeg Equalities/6  "r_ankle_roll"
  [r_ankle_pitch_ub] -> Mux4/2
  Mux/1 -> RLeg Equalities/1  "r_hip_pitch"
  Demux/5 -> [r_ankle_pitch]
  Demux2/6 -> [r_ankle_roll_lb]
  Demux/3 -> [r_hip_yaw]
  rLeg_lb/1 -> Demux2/1

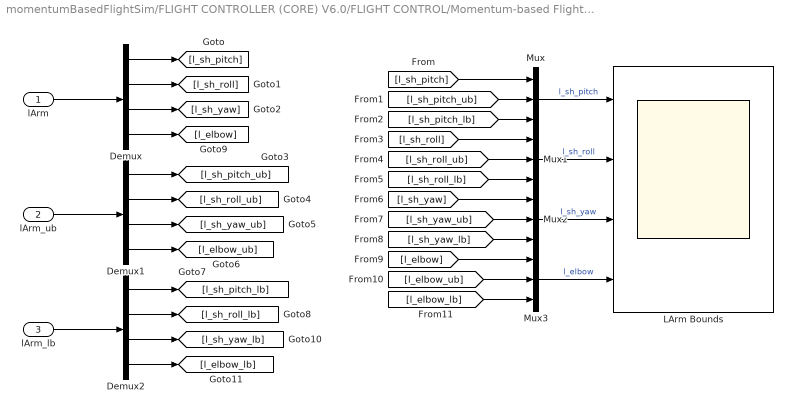
== system momentumBasedFlightSim/FLIGHT CONTROLLER (CORE) V6.0/FLIGHT CONTROL/Momentum-based Flight Control QP/Compute QP Quantities/Visualize QP Quantities/Input Boundaries/Vis LArm Bounds ==
  lArm : Inport
  lArm_ub : Inport  Port=2
  lArm_lb : Inport  Port=3
  Demux : Demux  Outputs=Config.N_ARMS/2
  Demux1 : Demux  Outputs=Config.N_ARMS/2
  Demux2 : Demux  Outputs=Config.N_ARMS/2
  LArm Bounds : Scope  NumInputPorts=4
  Mux{,1..3} (4 alike) : Mux  Inputs=3
  wires:
  [l_elbow_lb] -> Mux3/3
  [l_elbow_ub] -> Mux3/2
  [l_elbow] -> Mux3/1
  [l_sh_yaw_lb] -> Mux2/3
  [l_sh_yaw_ub] -> Mux2/2
  [l_sh_yaw] -> Mux2/1
  [l_sh_roll_lb] -> Mux1/3
  [l_sh_roll_ub] -> Mux1/2
  [l_sh_roll] -> Mux1/1
  [l_sh_pitch_lb] -> Mux/3
  [l_sh_pitch_ub] -> Mux/2
  [l_sh_pitch] -> Mux/1
  Mux3/1 -> LArm Bounds/4  "l_elbow"
  Demux2/4 -> [l_elbow_lb]
  Demux2/2 -> [l_sh_roll_lb]
  Demux2/3 -> [l_sh_yaw_lb]
  Demux2/1 -> [l_sh_pitch_lb]
  lArm_lb/1 -> Demux2/1
  lArm_ub/1 -> Demux1/1
  Demux1/2 -> [l_sh_roll_ub]
  Demux1/1 -> [l_sh_pitch_ub]
  Demux1/3 -> [l_sh_yaw_ub]
  Demux1/4 -> [l_elbow_ub]
  Demux/4 -> [l_elbow]
  lArm/1 -> Demux/1
  Demux/3 -> [l_sh_yaw]
  Demux/1 -> [l_sh_pitch]
  Mux1/1 -> LArm Bounds/2  "l_sh_roll"
  Demux/2 -> [l_sh_roll]
  Mux2/1 -> LArm Bounds/3  "l_sh_yaw"
  Mux/1 -> LArm Bounds/1  "l_sh_pitch"

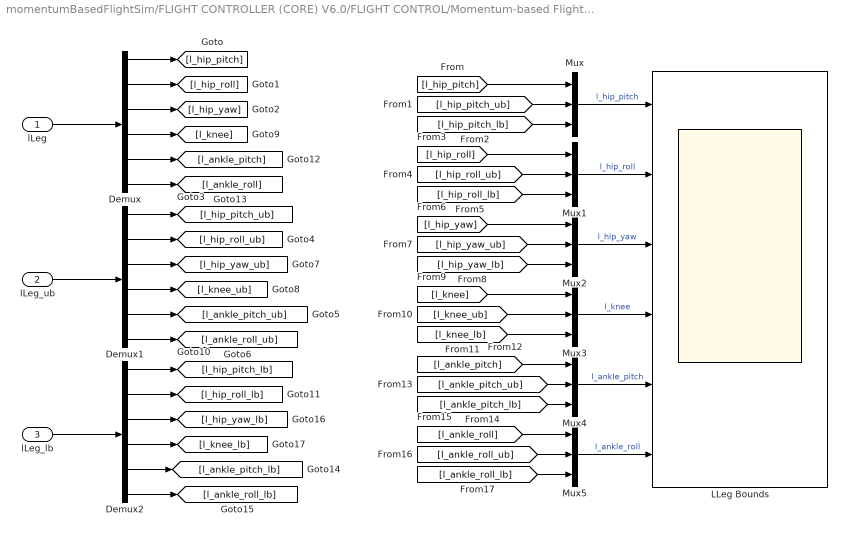
== system momentumBasedFlightSim/FLIGHT CONTROLLER (CORE) V6.0/FLIGHT CONTROL/Momentum-based Flight Control QP/Compute QP Quantities/Visualize QP Quantities/Input Boundaries/Vis LLeg Bounds ==
  lLeg : Inport
  lLeg_ub : Inport  Port=2
  lLeg_lb : Inport  Port=3
  Demux : Demux  Outputs=Config.N_LEGS/2
  Demux1 : Demux  Outputs=Config.N_LEGS/2
  Demux2 : Demux  Outputs=Config.N_LEGS/2
  LLeg Bounds : Scope  NumInputPorts=6
  Mux{,1..5} (6 alike) : Mux  Inputs=3
  wires:
  [l_ankle_roll_lb] -> Mux5/3
  [l_ankle_roll_ub] -> Mux5/2
  [l_ankle_roll] -> Mux5/1
  [l_ankle_pitch_lb] -> Mux4/3
  [l_ankle_pitch_ub] -> Mux4/2
  [l_ankle_pitch] -> Mux4/1
  [l_knee_lb] -> Mux3/3
  [l_knee_ub] -> Mux3/2
  [l_knee] -> Mux3/1
  [l_hip_yaw_lb] -> Mux2/3
  [l_hip_yaw_ub] -> Mux2/2
  [l_hip_yaw] -> Mux2/1
  [l_hip_roll_lb] -> Mux1/3
  [l_hip_roll_ub] -> Mux1/2
  [l_hip_roll] -> Mux1/1
  [l_hip_pitch_lb] -> Mux/3
  [l_hip_pitch_ub] -> Mux/2
  [l_hip_pitch] -> Mux/1
  Mux5/1 -> LLeg Bounds/6  "l_ankle_roll"
  Mux4/1 -> LLeg Bounds/5  "l_ankle_pitch"
  Demux2/4 -> [l_knee_lb]
  Demux2/3 -> [l_hip_yaw_lb]
  Demux2/1 -> [l_hip_pitch_lb]
  Demux2/2 -> [l_hip_roll_lb]
  Demux2/5 -> [l_ankle_pitch_lb]
  Demux2/6 -> [l_ankle_roll_lb]
  lLeg_lb/1 -> Demux2/1
  Demux1/1 -> [l_hip_pitch_ub]
  Demux1/2 -> [l_hip_roll_ub]
  Demux1/5 -> [l_ankle_pitch_ub]
  lLeg_ub/1 -> Demux1/1
  Demux1/6 -> [l_ankle_roll_ub]
  Demux1/4 -> [l_knee_ub]
  Demux1/3 -> [l_hip_yaw_ub]
  Demux/6 -> [l_ankle_roll]
  Demux/5 -> [l_ankle_pitch]
  Mux1/1 -> LLeg Bounds/2  "l_hip_roll"
  Mux2/1 -> LLeg Bounds/3  "l_hip_yaw"
  Demux/1 -> [l_hip_pitch]
  Demux/3 -> [l_hip_yaw]
  Mux3/1 -> LLeg Bounds/4  "l_knee"
  Demux/2 -> [l_hip_roll]
  Demux/4 -> [l_knee]
  lLeg/1 -> Demux/1
  Mux/1 -> LLeg Bounds/1  "l_hip_pitch"

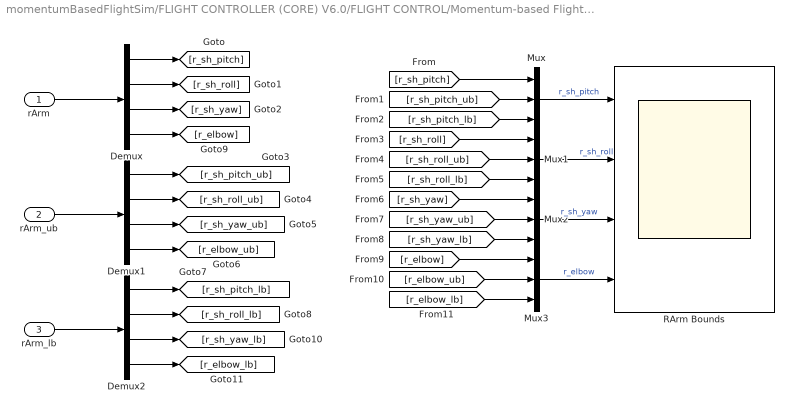
== system momentumBasedFlightSim/FLIGHT CONTROLLER (CORE) V6.0/FLIGHT CONTROL/Momentum-based Flight Control QP/Compute QP Quantities/Visualize QP Quantities/Input Boundaries/Vis RArm Bounds ==
  rArm : Inport
  rArm_ub : Inport  Port=2
  rArm_lb : Inport  Port=3
  Demux : Demux  Outputs=Config.N_ARMS/2
  Demux1 : Demux  Outputs=Config.N_ARMS/2
  Demux2 : Demux  Outputs=Config.N_ARMS/2
  Mux{,1..3} (4 alike) : Mux  Inputs=3
  RArm Bounds : Scope  NumInputPorts=4
  wires:
  Mux2/1 -> RArm Bounds/3  "r_sh_yaw"
  Demux2/3 -> [r_sh_yaw_lb]
  Demux/1 -> [r_sh_pitch]
  Demux1/2 -> [r_sh_roll_ub]
  Mux3/1 -> RArm Bounds/4  "r_elbow"
  [r_sh_pitch_ub] -> Mux/2
  Demux1/1 -> [r_sh_pitch_ub]
  [r_elbow] -> Mux3/1
  [r_sh_roll] -> Mux1/1
  Demux/3 -> [r_sh_yaw]
  Mux/1 -> RArm Bounds/1  "r_sh_pitch"
  [r_sh_roll_lb] -> Mux1/3
  Demux2/4 -> [r_elbow_lb]
  [r_sh_roll_ub] -> Mux1/2
  rArm_lb/1 -> Demux2/1
  Demux/4 -> [r_elbow]
  Demux1/4 -> [r_elbow_ub]
  Demux2/2 -> [r_sh_roll_lb]
  [r_sh_yaw] -> Mux2/1
  Demux1/3 -> [r_sh_yaw_ub]
  rArm_ub/1 -> Demux1/1
  Demux2/1 -> [r_sh_pitch_lb]
  Demux/2 -> [r_sh_roll]
  [r_elbow_ub] -> Mux3/2
  rArm/1 -> Demux/1
  [r_elbow_lb] -> Mux3/3
  [r_sh_pitch_lb] -> Mux/3
  Mux1/1 -> RArm Bounds/2  "r_sh_roll"
  [r_sh_pitch] -> Mux/1
  [r_sh_yaw_lb] -> Mux2/3
  [r_sh_yaw_ub] -> Mux2/2

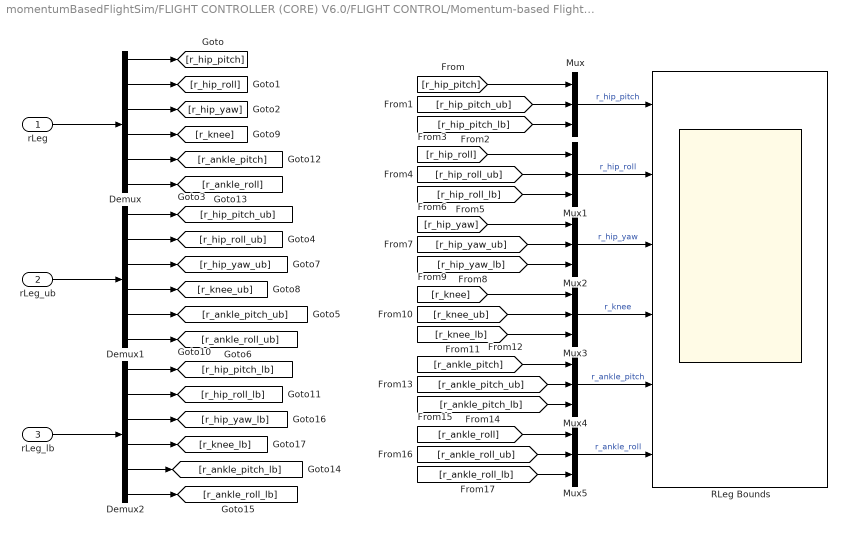
== system momentumBasedFlightSim/FLIGHT CONTROLLER (CORE) V6.0/FLIGHT CONTROL/Momentum-based Flight Control QP/Compute QP Quantities/Visualize QP Quantities/Input Boundaries/Vis RLeg Bounds ==
  rLeg : Inport
  rLeg_ub : Inport  Port=2
  rLeg_lb : Inport  Port=3
  Demux : Demux  Outputs=Config.N_LEGS/2
  Demux1 : Demux  Outputs=Config.N_LEGS/2
  Demux2 : Demux  Outputs=Config.N_LEGS/2
  Mux{,1..5} (6 alike) : Mux  Inputs=3
  RLeg Bounds : Scope  NumInputPorts=6
  wires:
  Demux/2 -> [r_hip_roll]
  Demux1/4 -> [r_knee_ub]
  Mux2/1 -> RLeg Bounds/3  "r_hip_yaw"
  Demux1/2 -> [r_hip_roll_ub]
  Demux1/5 -> [r_ankle_pitch_ub]
  [r_ankle_pitch_lb] -> Mux4/3
  [r_hip_yaw_lb] -> Mux2/3
  Demux1/6 -> [r_ankle_roll_ub]
  [r_hip_roll] -> Mux1/1
  Demux1/3 -> [r_hip_yaw_ub]
  Demux1/1 -> [r_hip_pitch_ub]
  [r_ankle_pitch] -> Mux4/1
  Demux/1 -> [r_hip_pitch]
  [r_knee] -> Mux3/1
  Demux/4 -> [r_knee]
  Mux4/1 -> RLeg Bounds/5  "r_ankle_pitch"
  [r_hip_pitch] -> Mux/1
  Demux2/5 -> [r_ankle_pitch_lb]
  Demux2/3 -> [r_hip_yaw_lb]
  Demux2/2 -> [r_hip_roll_lb]
  [r_ankle_roll_lb] -> Mux5/3
  [r_hip_yaw_ub] -> Mux2/2
  [r_hip_yaw] -> Mux2/1
  [r_hip_pitch_lb] -> Mux/3
  Demux/6 -> [r_ankle_roll]
  rLeg/1 -> Demux/1
  Demux2/1 -> [r_hip_pitch_lb]
  [r_knee_lb] -> Mux3/3
  Mux3/1 -> RLeg Bounds/4  "r_knee"
  Mux1/1 -> RLeg Bounds/2  "r_hip_roll"
  Demux2/4 -> [r_knee_lb]
  [r_knee_ub] -> Mux3/2
  [r_ankle_roll] -> Mux5/1
  [r_hip_roll_lb] -> Mux1/3
  [r_hip_roll_ub] -> Mux1/2
  [r_ankle_roll_ub] -> Mux5/2
  rLeg_ub/1 -> Demux1/1
  [r_hip_pitch_ub] -> Mux/2
  Mux5/1 -> RLeg Bounds/6  "r_ankle_roll"
  [r_ankle_pitch_ub] -> Mux4/2
  Mux/1 -> RLeg Bounds/1  "r_hip_pitch"
  Demux/5 -> [r_ankle_pitch]
  Demux2/6 -> [r_ankle_roll_lb]
  Demux/3 -> [r_hip_yaw]
  rLeg_lb/1 -> Demux2/1

== system momentumBasedFlightSim/FLIGHT CONTROLLER (CORE) V6.0/FLIGHT CONTROL/Momentum-based Flight Control QP/Compute QP Quantities/Visualize QP Quantities/Input Boundaries/Vis Torso Bounds ==
  torso : Inport
  torso_ub : Inport  Port=2
  torso_lb : Inport  Port=3
  Demux : Demux  Outputs=Config.N_TORSO
  Demux1 : Demux  Outputs=Config.N_TORSO
  Demux2 : Demux  Outputs=Config.N_TORSO
  Mux : Mux  Inputs=3
  Mux1 : Mux  Inputs=3
  Mux2 : Mux  Inputs=3
  Torso Bounds : Scope  NumInputPorts=3
  wires:
  Mux1/1 -> Torso Bounds/2  "torso_roll"
  Mux2/1 -> Torso Bounds/3  "torso_yaw"
  Mux/1 -> Torso Bounds/1  "torso_pitch"
  [torso_yaw_lb] -> Mux2/3
  [torso_yaw_ub] -> Mux2/2
  [torso_yaw] -> Mux2/1
  [torso_roll] -> Mux1/1
  [torso_roll_ub] -> Mux1/2
  [torso_roll_lb] -> Mux1/3
  [torso_pitch_lb] -> Mux/3
  [torso_pitch_ub] -> Mux/2
  [torso_pitch] -> Mux/1
  Demux2/3 -> [torso_yaw_lb]
  Demux2/2 -> [torso_roll_lb]
  Demux2/1 -> [torso_pitch_lb]
  Demux1/3 -> [torso_yaw_ub]
  Demux1/1 -> [torso_pitch_ub]
  Demux1/2 -> [torso_roll_ub]
  Demux/3 -> [torso_yaw]
  Demux/2 -> [torso_roll]
  Demux/1 -> [torso_pitch]
  torso_lb/1 -> Demux2/1
  torso_ub/1 -> Demux1/1
  torso/1 -> Demux/1

== matlab function momentumBasedFlightSim/FLIGHT CONTROLLER (CORE) V6.0/FLIGHT CONTROL/Flight 0 Reference Generator/Compute Gains And References/Online Planner/Flight Planner - CoM and Base ==
  data: posCoM_des output; accCoM_gravity_ref output; rot_vel_acc_jerk_base_des output; time input; posCoM_0 input; w_R_b_0 input; Config parameter
function [posCoM_des, accCoM_gravity_ref, rot_vel_acc_jerk_base_des] = onlineFlightPlannerCoM_and_Base_FCN(time, posCoM_0, w_R_b_0, Config)

    [posCoM_des, accCoM_gravity_ref, rot_vel_acc_jerk_base_des] = onlineFlightPlannerCoM_and_Base(time, posCoM_0, w_R_b_0, Config);
end

== matlab function momentumBasedFlightSim/FLIGHT CONTROLLER (CORE) V6.0/FLIGHT CONTROL/Flight 0 Reference Generator/Compute Gains And References/Online Planner/Flight Planner - Joints and Thrusts ==
  data: accCoM_des input; m input; jointPos_0 input; Aj0 input; jetsIntensities_des output; jointPos_des output; Config parameter
function [jetsIntensities_des, jointPos_des] = onlineFlightPlannerJoints_and_ThrustFCN(accCoM_des, m, jointPos_0, Aj0, Config)

[jetsIntensities_des, jointPos_des] = onlineFlightPlannerJoints_and_Thrust(accCoM_des, m, jointPos_0, Aj0, Config);

end

== matlab function momentumBasedFlightSim/FLIGHT CONTROLLER (CORE) V6.0/FLIGHT CONTROL/Flight 0 Reference Generator/Compute Gains And References/Online Planner/Smooth CoM References/Combine CoM References ==
  data: CoM_pos input; CoM_vel input; CoM_acc input; CoM_acc_gravity input; pos_vel_acc_jerk_CoM_des output
function pos_vel_acc_jerk_CoM_des = combineCoMRef(CoM_pos, CoM_vel, CoM_acc, CoM_acc_gravity)

% composing the CoM references. The reference acceleration has to sum up
% with the gravity-compensation reference that is necessary for balancing
pos_vel_acc_jerk_CoM_des = [CoM_pos, CoM_vel, (CoM_acc + CoM_acc_gravity), zeros(3,1)];

% WARNING: jerk ref is set to zero by default!

end

== matlab function momentumBasedFlightSim/FLIGHT CONTROLLER (CORE) V6.0/FLIGHT CONTROL/Flight 0 Reference Generator/Take Off//Landing State Detector/MATLAB Function ==
  data: wrench_l input; feetContactIsActive output; wrench_r input; Config parameter; robotIsLanded output; oneFootIsInContact output
function [feetContactIsActive, robotIsLanded, oneFootIsInContact] = feetContactActivationFCN(wrench_l, wrench_r, Config)

    [feetContactIsActive, robotIsLanded, oneFootIsInContact] = iRonCubLib.feetContactActivation(wrench_l, wrench_r, Config);
end

== matlab function momentumBasedFlightSim/Jets Feedback Lin. Control/Filter JetDerivative Desired ==
  data: jetIntensitiesEst input; jetIntensitiesDerivativeDes input; jetIntensitiesDerivativeDes output; Config parameter
function jetIntensitiesDerivativeDes = filterIntensitiesDerivativeFCN(jetIntensitiesEst, jetIntensitiesDerivativeDes, Config)

jetIntensitiesDerivativeDes = filterIntensitiesDerivative(jetIntensitiesEst, jetIntensitiesDerivativeDes, Config);
end

== matlab function momentumBasedFlightSim/Online Visualizer/Get RPY from rotation matrix ==
  data: w_R_b input; rollPitchYaw output
function rollPitchYaw = rollPitchYawFromRotationFCN(w_R_b)

rollPitchYaw = wbc.rollPitchYawFromRotation(w_R_b);

end

== matlab function momentumBasedFlightSim/Online Visualizer/MATLAB Function2 ==
  data: RPY_Corr output; rollPitchYaw input
function RPY_Corr = correctYawAngleFCN(rollPitchYaw)

    RPY_Corr = correctYawAngle(rollPitchYaw);

end

== matlab function momentumBasedFlightSim/FLIGHT CONTROLLER (CORE) V6.0/FLIGHT CONTROL/Momentum-based Flight Control QP/Compute QP Quantities/Flight 0 Control with QP ==
  data: posCoM_error input; HessianQP output; jointPos input; w_baseTwist input; jetsIntensities input; J_jets input; J_CoM input; w_R_b input; matrixOfJetsAxes input; matrixOfJetsArms input; M input; L input; CMM input; w_I_c input; pos_vel_acc_jerk_CoM_des input; rot_vel_acc_jerk_base_des input; jointPos_des input; jetsIntensities_des input; KP_momentum input; KD_momentum input; KP_postural input; u_star input; gradientQP output; lb output; ub output; A_equality output; lbA output; ubA output; costVectorQP output; LDot_estimated output; LDot_tilde output; L_tilde output; intL_tilde output; jetsIntensitiesDot_postural output; Config parameter
function [HessianQP, gradientQP, lb, ub, A_equality, lbA, ubA, costVectorQP, LDot_estimated, LDot_tilde, L_tilde, intL_tilde, jetsIntensitiesDot_postural] = ...
             flightControl_0_QP_experiments_v3(posCoM_error, jointPos, w_baseTwist, jetsIntensities, J_jets, J_CoM, w_R_b, matrixOfJetsAxes, matrixOfJetsArms, M, L, CMM, ...
                                               w_I_c, pos_vel_acc_jerk_CoM_des, rot_vel_acc_jerk_base_des, jointPos_des, jetsIntensities_des, KP_momentum, KD_momentum, KP_postural, u_star, Config)

          [HessianQP, gradientQP, lb, ub, A_equality, lbA, ubA, costVectorQP, LDot_estimated, LDot_tilde, L_tilde, intL_tilde, jetsIntensitiesDot_postural] = ...
              flightControl_0_QP_experiments_v3(posCoM_error, jointPos, w_baseTwist, jetsIntensities, J_jets, J_CoM, w_R_b, matrixOfJetsAxes, matrixOfJetsArms, M, L, CMM, ...
                                                w_I_c, pos_vel_acc_jerk_CoM_des, rot_vel_acc_jerk_base_des, jointPos_des, jetsIntensities_des, KP_momentum, KD_momentum, KP_postural, u_star, Config);
end

== matlab function momentumBasedFlightSim/FLIGHT CONTROLLER (CORE) V6.0/FLIGHT CONTROL/Momentum-based Flight Control QP/Compute QP Quantities/Integrate CoM Velocity/Get CoM Position Error from Integral but Only in Hovering/Get CoM initial condition ==
  data: feetContactIsActive input; error_posCoM input; error_posCoM_0 output
function error_posCoM_0 = resetInitialCondition_CoMError(feetContactIsActive, error_posCoM)

persistent feetContact_prev error_posCoM_updated

if isempty(error_posCoM_updated)

    error_posCoM_updated = error_posCoM;
end
if isempty(feetContact_prev)

    feetContact_prev = feetContactIsActive;
end

if abs(feetContact_prev - feetContactIsActive) > 0.5

    error_posCoM_updated = error_posCoM;
    feetContact_prev = feetContactIsActive;
end

error_posCoM_0 = error_posCoM_updated;

== matlab function momentumBasedFlightSim/FLIGHT CONTROLLER (CORE) V6.0/FLIGHT CONTROL/Momentum-based Flight Control QP/Compute QP Quantities/Integrate CoM Velocity/Select CoM Pos Error/Select CoM Pos Error ==
  data: posCoM_error_fromInt_HoveringOnly input; posCoM_error_fromIntegral input; posCoM_error_fromKinematics input; posCoM_error output; Config parameter
function posCoM_error = selectCoMPosErrorFCN(posCoM_error_fromInt_HoveringOnly, posCoM_error_fromIntegral, posCoM_error_fromKinematics, Config)

    posCoM_error = iRonCubLib.selectCoMPosError(posCoM_error_fromInt_HoveringOnly, posCoM_error_fromIntegral, posCoM_error_fromKinematics, Config);
end

== matlab function momentumBasedFlightSim/FLIGHT CONTROLLER (CORE) V6.0/FLIGHT CONTROL/Momentum-based Flight Control QP/Filtering and Saturations/Filters on jointVel/joint_vel_saturation ==
  data: jointPos input; jointVel_des input size=[Config.N_DOF,1]; JetState input; jointVel output size=[Config.N_DOF,1]; Config parameter
function jointVel = saturateJointsVelocity(jointPos, jointVel_des, JetState, Config)
    jointVel = saturateJointsVelocity(jointPos, jointVel_des, JetState, Config);
end

== matlab function momentumBasedFlightSim/FLIGHT CONTROLLER (CORE) V6.0/FLIGHT CONTROL/Compute Global CoP/Compute global CoP ==
  data: wrench_left input; global_cop output; wrench_right input; H_left input; H_right input; robotOnGround output
function [global_cop, robotOnGround] = compute_global_cop(wrench_left, wrench_right, H_left, H_right)
[global_cop, robotOnGround] = compute_global_cop(wrench_left, wrench_right, H_left, H_right);

== matlab function momentumBasedFlightSim/FLIGHT CONTROLLER (CORE) V6.0/Failure Detection/Turbines Failure Detection ==
  data: jetsIntensities input; turbineStatus output; jetsIntensities_star input; t input; Config parameter; T_err_avg output; T_err output
function [turbineStatus, T_err_avg, T_err] = turbinesFailureDetectorFCN(jetsIntensities, jetsIntensities_star, t, Config)

    [turbineStatus, T_err_avg, T_err] = turbinesFailureDetector(jetsIntensities, jetsIntensities_star, t, Config);
end

== matlab function momentumBasedFlightSim/FLIGHT CONTROLLER (CORE) V6.0/FLIGHT CONTROL/Flight 0 Reference Generator/Compute Gains And References/Compute Gains/Diagonalize ==
  data: k input; K output
function K = diagonalMatrixFromVectorFCN(k)

    K = wbc.diagonalMatrixFromVector(k);
end

== matlab function momentumBasedFlightSim/FLIGHT CONTROLLER (CORE) V6.0/FLIGHT CONTROL/Flight 0 Reference Generator/Compute Gains And References/Compute Gains/Diagonalize1 ==
  data: k input; K output
function K = diagonalMatrixFromVectorFCN(k)

    K = wbc.diagonalMatrixFromVector(k);
end

== matlab function momentumBasedFlightSim/FLIGHT CONTROLLER (CORE) V6.0/FLIGHT CONTROL/Flight 0 Reference Generator/Compute Gains And References/Compute Gains/Diagonalize2 ==
  data: k input; K output
function K = diagonalMatrixFromVectorFCN(k)

    K = wbc.diagonalMatrixFromVector(k);
end

== matlab function momentumBasedFlightSim/FLIGHT CONTROLLER (CORE) V6.0/FLIGHT CONTROL/Flight 0 Reference Generator/Compute Gains And References/Online Planner/Compute matrix Aj ==
  data: Aj output; matrixOfJetsAxes input; matrixOfJetsArms input
function Aj = computeMatrixAj_momentumFCN(matrixOfJetsAxes, matrixOfJetsArms)

Aj = computeMatrixAj_momentum(matrixOfJetsAxes, matrixOfJetsArms);
end
